simulink model "MPC_NN"  (R2022a)
settings: Solver=VariableStepAuto  StartTime=0.0  StopTime=40  FixedStep=0.01  RelTol=1e-3
undefined symbols (not defined in the file or in its folder): neural_Nc, neural_Np, neural_Qy, neural_R, sigbuilder_block
libraries: autolibutils x8, autolibshared x6, vehdynlibviscommon x2, simulink x2
(part 4 of 4)

== system MPC_NN/Subsystem2/Powertrain & Driveline/Driveline/RWD ==
  TPowertrain : Inport
  RWD : Gain  Gain=[0;0;1;1]
  TAxles : Outport  VectorParamsAs1DForOutWhenUnconnected=off
  wires:
  TPowertrain/1 -> RWD/1
  RWD/1 -> TAxles/1

== matlab function MPC_NN/Neural Network/MATLAB Function2 ==
  data: nc input; np input; Np output
function Np = fcn(nc,np)

np = round(np);
if np<9
    np = 9;
end
if np < nc
    np = nc + 3;
end
Np=np;

== matlab function MPC_NN/Neural Network/MATLAB Function3 ==
  data: qy input; Qy output
function Qy = fcn(qy)

if qy<0.75
    qy = 0.75;
end
if qy >10
qy=10;
end

Qy=qy;

== matlab function MPC_NN/Neural Network/MATLAB Function4 ==
  data: r input; R output
function R = fcn(r)

if r<0.01
    r = 0.01;
end
if r>0.5
r=0.5;
end

R=r;

== matlab function MPC_NN/Subsystem1/MPC1 ==
  settings: updateMethod=DISCRETE
  data: u output; Vx input; u input; y input; r input; m input; Iz input; lf input; lr input; Cf input; Cr input; dt input; a input; N input; Nc input; Np input; Qy input; R input; u_min input; u_max input; deltau_min input; deltau_max input; y_min input; y_max input; xm input
function u = fcn(Vx, u,y,r,m,Iz,lf,lr,Cf,Cr,dt,a,N,Nc,Np,Qy,R,u_min,u_max,deltau_min,deltau_max,y_min,y_max,xm)

tic;

coder.extrinsic('c2dm')
%coder.extrinsic(function)

%load('new_trajectory.mat')


% Model identification

% m = 1575;
% Iz = 2875;
% lf = 1.2;
% lr = 1.6;
% Cf = 19000;
% Cr = 33000;


%state vector  [y_dot phi phi_dot y]
Ac = [-(2*Cf+2*Cr)/m/Vx, 0, -Vx-(2*Cf*lf-2*Cr*lr)/m/Vx, 0;
     0, 0, 1, 0;
     -(2*Cf*lf-2*Cr*lr)/Iz/Vx, 0, -(2*Cf*lf^2+2*Cr*lr^2)/Iz/Vx, 0;
     1, Vx, 0, 0];
Bc = [2*Cf/m 0 2*Cf*lf/Iz 0]';   
Cc = [0 0 0 1];
%C2 = [0 0 0 1; 0 1 0 0];
Dc = zeros(1,1);

%dt=0.1;
[Ad, Bd, Cd, Dd]=c2dm(Ac,Bc,Cc,Dc,dt,'zoh');
% tic
% Make the augmented state-space model
n1 = 0;
m1 = 0;
n_in = 0;

[m1, n1] = size(Cd);
[n1, n_in] = size(Bd);
A = eye(n1+m1, n1+m1);
A(1:n1, 1:n1) = Ad;
A(n1+1:n1+m1,1:n1) = Cd*Ad;
B = zeros(n1+m1, n_in);
B(1:n1,:) = Bd;
B(n1+1:n1+m1,:) = Cd*Bd;
C = zeros(m1, n1+m1);
C(:, n1+1:n1+m1) = eye(m1, m1);
D = Dd;


% a=0.5;
% Nc=5;
% N=5; %you can increase N
% Np=25;

%obtain constraints data matrices

[M1,Lzerot]=Mdu(a,N,1,Nc);
M0=Mu(a,N,1,Nc);

%initial conditions for closed-loop simulation using constrained control
%specify the limits for ?u and u

%xm=zeros(n1,1);
% persistent xm;
% if isempty(xm)
%   xm=zeros(n1,1);
% end


persistent xm_old
if isempty(xm_old)
  %xm_old=[0; 0; 0; 37];
  xm_old=zeros(4,1);
end


persistent Xf
if isempty(Xf)
  Xf=[xm; y-r];
end


Xf=[xm-xm_old;y-r];
%end
xm_old=xm;

%specify constraints limits

% u_min=-pi/6;
% u_max=pi/6;
% deltau_min=-pi/12;
% deltau_max=pi/12;
% 
%  y_min=-2;
%  y_max=6;
y_bar_min=y_min-r;
y_bar_max=y_max-r;


%up=0.0;
up=u;

% C2 = [0 0 0 1; 0 1 0 0];
% Cc = [0 0 0 1];
% Generate matrices required for the predictive control cost function J

% Q=C'*C;
% R=0.0001;
Q=[0,0,0,0,0;0,0,0,0,0;0,0,0,0,0;0,0,0,0,0;0,0,0,0,Qy];


%for kk=1:N_sim-1;
% Continuous-time model

% Ac = [-(2*Cf+2*Cr)/m, 0, -Vx-(2*Cf*lf-2*Cr*lr)/(m*Vx), 0;
%      0, 0, 1, 0;
%      -(2*Cf*lf-2*Cr*lr)/Iz/Vx, 0, -(2*Cf*lf^2+2*Cr*lr^2)/Iz/Vx, 0;
%      1, Vx, 0, 0];
% Bc = [2*Cf/m 0 2*Cf*lf/Iz 0]';   
% Cc = [0 0 0 1];
% C2 = [0 0 0 1; 0 1 0 0];
% Dc = zeros(1,1);

% Minimal realisation

% [num,den] = ss2tf(Ac,Bc,Cc,Dc);
% Gs = tf(num,den);
% 
% Gsmin=ss(Gs,'min');
% [Am,Bm,Cm,Dm]=ssdata(Gsmin);

% Discrete-time model

% dt=0.1;
% [Ad, Bd, Cd, Dd]=c2dm(Ac,Bc,Cc,Dc,dt,'zoh');

% Make the augmented state-space model

% [m1, n1] = size(Cd);
% [n1, n_in] = size(Bd);
% A = eye(n1+m1, n1+m1);
% A(1:n1, 1:n1) = Ad;
% A(n1+1:n1+m1,1:n1) = Cd*Ad;
% B = zeros(n1+m1, n_in);
% B(1:n1,:) = Bd;
% B(n1+1:n1+m1,:) = Cd*Bd;
% C = zeros(m1, n1+m1);
% C(:, n1+1:n1+m1) = eye(m1, m1);
% D = Dd;



[Phi,F]=mpcgain(Ad,Bd,Cd,N,Np);
[Omega,Psi]=dmpc(A,B,a,N,Np,Q,R);







%% constrains on U first
 M=[M0;-M0;M1;-M1;Phi(1:Nc,1)*Lzerot;-Phi(1:Nc,1)*Lzerot];


%closed-loop simulation performed recursively
%optimal control is also found recursively

%% constrains on u first
gamma=[(u_max-up)*ones(Nc,1);(-u_min+up)*ones(Nc,1);...
    deltau_max*ones(Nc,1);-deltau_min*ones(Nc,1);...
    y_bar_max-F(1:Nc,:)*Xf;-y_bar_min+F(1:Nc,:)*Xf];

eta=QPhild(Omega,Psi*Xf,M,gamma);

deltau=Lzerot*eta;
if (deltau>deltau_max) deltau=deltau_max;end
if (deltau<deltau_min) deltau=deltau_min;end
u=u+deltau;
if (u>u_max) deltau=u_max-up; u=u_max; end
if (u<u_min) deltau=u_min-up; u=u_min; end


%deltau1(1,kk)=deltau; %save data
%u1(1,kk)=u; %save data
%y1(:,kk)=y; %save data

%%%%
%plant simulation
%%%%%%


% xm=Ad*xm+Bd*u; % calculate xm(k+1)
% y=Cd*xm; %calculate y(k+1)
% y2=C2*xm;
% y3(1,kk)=y2(2,1);
% Xf=[xm-xm_old;y-r(1,kk)];
% y_bar_min=y_min-r(1,kk);
% y_bar_max=y_max-r(1,kk);

%timeElapsed = toc

== matlab function MPC_NN/Subsystem2/MPC ==
  settings: updateMethod=DISCRETE
  data: u output; Vx input; u input; y input; r input; m input; Iz input; lf input; lr input; Cf input; Cr input; dt input; a input; N input; Nc input; Np input; Qy input; R input; u_min input; u_max input; deltau_min input; deltau_max input; y_min input; y_max input; xm input
function u = fcn(Vx, u,y,r,m,Iz,lf,lr,Cf,Cr,dt,a,N,Nc,Np,Qy,R,u_min,u_max,deltau_min,deltau_max,y_min,y_max,xm)

tic;

coder.extrinsic('c2dm')
%coder.extrinsic(function)

%load('new_trajectory.mat')


% Model identification

% m = 1575;
% Iz = 2875;
% lf = 1.2;
% lr = 1.6;
% Cf = 19000;
% Cr = 33000;


%state vector  [y_dot phi phi_dot y]
Ac = [-(2*Cf+2*Cr)/m/Vx, 0, -Vx-(2*Cf*lf-2*Cr*lr)/m/Vx, 0;
     0, 0, 1, 0;
     -(2*Cf*lf-2*Cr*lr)/Iz/Vx, 0, -(2*Cf*lf^2+2*Cr*lr^2)/Iz/Vx, 0;
     1, Vx, 0, 0];
Bc = [2*Cf/m 0 2*Cf*lf/Iz 0]';   
Cc = [0 0 0 1];
%C2 = [0 0 0 1; 0 1 0 0];
Dc = zeros(1,1);

%dt=0.1;
[Ad, Bd, Cd, Dd]=c2dm(Ac,Bc,Cc,Dc,dt,'zoh');
% tic
% Make the augmented state-space model
n1 = 0;
m1 = 0;
n_in = 0;

[m1, n1] = size(Cd);
[n1, n_in] = size(Bd);
A = eye(n1+m1, n1+m1);
A(1:n1, 1:n1) = Ad;
A(n1+1:n1+m1,1:n1) = Cd*Ad;
B = zeros(n1+m1, n_in);
B(1:n1,:) = Bd;
B(n1+1:n1+m1,:) = Cd*Bd;
C = zeros(m1, n1+m1);
C(:, n1+1:n1+m1) = eye(m1, m1);
D = Dd;


% a=0.5;
% Nc=5;
% N=5; %you can increase N
% Np=25;

%obtain constraints data matrices

[M1,Lzerot]=Mdu(a,N,1,Nc);
M0=Mu(a,N,1,Nc);

%initial conditions for closed-loop simulation using constrained control
%specify the limits for ?u and u

%xm=zeros(n1,1);
% persistent xm;
% if isempty(xm)
%   xm=zeros(n1,1);
% end


persistent xm_old
if isempty(xm_old)
  %xm_old=[0; 0; 0; 37];
  xm_old=zeros(4,1);
end


persistent Xf
if isempty(Xf)
  Xf=[xm; y-r];
end


Xf=[xm-xm_old;y-r];
%end
xm_old=xm;

%specify constraints limits

% u_min=-pi/6;
% u_max=pi/6;
% deltau_min=-pi/12;
% deltau_max=pi/12;
% 
%  y_min=-2;
%  y_max=6;
y_bar_min=y_min-r;
y_bar_max=y_max-r;


%up=0.0;
up=u;

% C2 = [0 0 0 1; 0 1 0 0];
% Cc = [0 0 0 1];
% Generate matrices required for the predictive control cost function J

% Q=C'*C;
% R=0.0001;
Q=[0,0,0,0,0;0,0,0,0,0;0,0,0,0,0;0,0,0,0,0;0,0,0,0,Qy];


%for kk=1:N_sim-1;
% Continuous-time model

% Ac = [-(2*Cf+2*Cr)/m, 0, -Vx-(2*Cf*lf-2*Cr*lr)/(m*Vx), 0;
%      0, 0, 1, 0;
%      -(2*Cf*lf-2*Cr*lr)/Iz/Vx, 0, -(2*Cf*lf^2+2*Cr*lr^2)/Iz/Vx, 0;
%      1, Vx, 0, 0];
% Bc = [2*Cf/m 0 2*Cf*lf/Iz 0]';   
% Cc = [0 0 0 1];
% C2 = [0 0 0 1; 0 1 0 0];
% Dc = zeros(1,1);

% Minimal realisation

% [num,den] = ss2tf(Ac,Bc,Cc,Dc);
% Gs = tf(num,den);
% 
% Gsmin=ss(Gs,'min');
% [Am,Bm,Cm,Dm]=ssdata(Gsmin);

% Discrete-time model

% dt=0.1;
% [Ad, Bd, Cd, Dd]=c2dm(Ac,Bc,Cc,Dc,dt,'zoh');

% Make the augmented state-space model

% [m1, n1] = size(Cd);
% [n1, n_in] = size(Bd);
% A = eye(n1+m1, n1+m1);
% A(1:n1, 1:n1) = Ad;
% A(n1+1:n1+m1,1:n1) = Cd*Ad;
% B = zeros(n1+m1, n_in);
% B(1:n1,:) = Bd;
% B(n1+1:n1+m1,:) = Cd*Bd;
% C = zeros(m1, n1+m1);
% C(:, n1+1:n1+m1) = eye(m1, m1);
% D = Dd;



[Phi,F]=mpcgain(Ad,Bd,Cd,N,Np);
[Omega,Psi]=dmpc(A,B,a,N,Np,Q,R);







%% constrains on U first
 M=[M0;-M0;M1;-M1;Phi(1:Nc,1)*Lzerot;-Phi(1:Nc,1)*Lzerot];


%closed-loop simulation performed recursively
%optimal control is also found recursively

%% constrains on u first
gamma=[(u_max-up)*ones(Nc,1);(-u_min+up)*ones(Nc,1);...
    deltau_max*ones(Nc,1);-deltau_min*ones(Nc,1);...
    y_bar_max-F(1:Nc,:)*Xf;-y_bar_min+F(1:Nc,:)*Xf];

eta=QPhild(Omega,Psi*Xf,M,gamma);

deltau=Lzerot*eta;
if (deltau>deltau_max) deltau=deltau_max;end
if (deltau<deltau_min) deltau=deltau_min;end
u=u+deltau;
if (u>u_max) deltau=u_max-up; u=u_max; end
if (u<u_min) deltau=u_min-up; u=u_min; end


%deltau1(1,kk)=deltau; %save data
%u1(1,kk)=u; %save data
%y1(:,kk)=y; %save data

%%%%
%plant simulation
%%%%%%


% xm=Ad*xm+Bd*u; % calculate xm(k+1)
% y=Cd*xm; %calculate y(k+1)
% y2=C2*xm;
% y3(1,kk)=y2(2,1);
% Xf=[xm-xm_old;y-r(1,kk)];
% y_bar_min=y_min-r(1,kk);
% y_bar_max=y_max-r(1,kk);

%timeElapsed = toc

== matlab function MPC_NN/Neural Network/MATLAB Function1 ==
  data: nc input; Nc output
function Nc = fcn(nc)

nc = round(nc);
if nc<5
    nc = 5;
end
Nc=nc;
